simulink model "Attitude_Controller"  (R2016b)
settings: Solver=VariableStepAuto  StartTime=0.0  StopTime=3  MaxStep=0.001  RelTol=1e-3
settings Model: Creator=Administrator  LastModifiedBy=Administrator

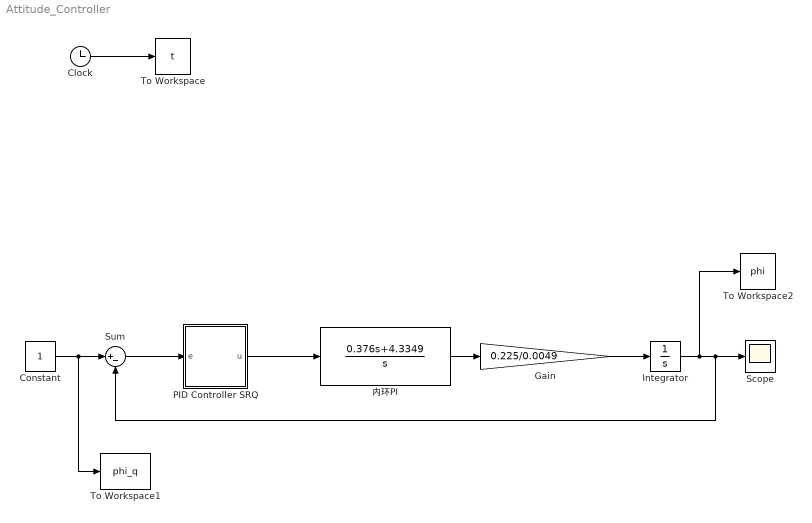
== system Attitude_Controller ==
  Clock : Clock
  Constant : Constant
  Gain : Gain  Gain=0.225/0.0049
  Integrator : Integrator
  PID Controller SRQ : Subsystem
  Scope : Scope
  Sum : Sum  Inputs=|+-
  To Workspace : ToWorkspace  VariableName=t  SampleTime=-1
  To Workspace1 : ToWorkspace  VariableName=phi_q  SampleTime=-1
  To Workspace2 : ToWorkspace  VariableName=phi  SampleTime=-1
  内环PI : TransferFcn  Numerator=[0.376 4.3349]  Denominator=[1 0]
  wires:
  Constant/1 -> To Workspace1/1, Sum/1
  PID Controller SRQ/1(u) -> 内环PI/1
  内环PI/1 -> Gain/1
  Gain/1 -> Integrator/1
  Integrator/1 -> To Workspace2/1, Sum/2, Scope/1
  Clock/1 -> To Workspace/1
  Sum/1 -> PID Controller SRQ/1(e)

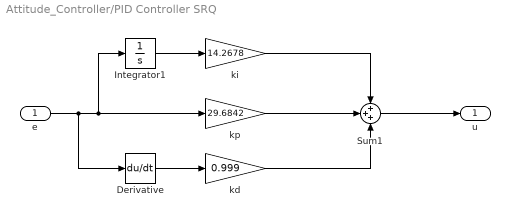
== system Attitude_Controller/PID Controller SRQ ==
  e : Inport
  Derivative : Derivative
  Integrator1 : Integrator
  Sum1 : Sum  Inputs=+++
  kd : Gain  Gain=0.999
  ki : Gain  Gain=14.2678
  kp : Gain  Gain=29.6842
  u : Outport
  wires:
  Sum1/1 -> u/1
  Integrator1/1 -> ki/1
  kd/1 -> Sum1/3
  kp/1 -> Sum1/2
  e/1 -> Derivative/1, Integrator1/1, kp/1
  Derivative/1 -> kd/1
  ki/1 -> Sum1/1
